simulink model "roll_1dof_model"  (R2024b)
settings: Solver=ode45  StartTime=0.0  StopTime=sim_stopTime  RelTol=1e-3
undefined symbols (not defined in the file): command_rollStep, command_stepTime, controller_inner_Kp, controller_outer_Kp, controller_outer_maxRateCmd, fin_actuatorTau, fin_maxDeflection, fin_maxRate, roll_design_Ixx, roll_design_p, roll_design_phi, roll_Ldelta, roll_Lp, sensor_attitudeTau, sensor_gyroTau
settings Model: Creator=kiwamoto  LastModifiedBy=kohei
settings ModelReferenceCC: UpdateModelReferenceTargets=IfOutOfDate

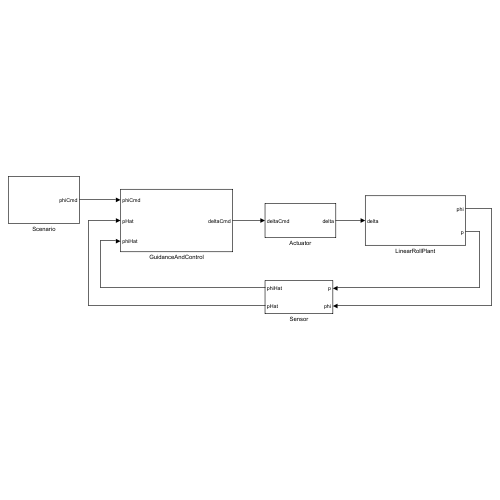
[thumbnail: Simulink's stored preview of the top-level diagram]
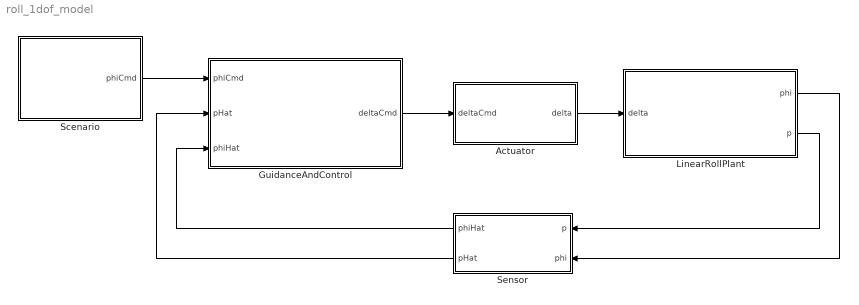
== system roll_1dof_model ==
  Actuator : Subsystem
  GuidanceAndControl : Subsystem
  LinearRollPlant : Subsystem
  Scenario : Subsystem
  Sensor : Subsystem
  wires:
  Scenario/1(phiCmd) -> GuidanceAndControl/1(phiCmd)
  GuidanceAndControl/1(deltaCmd) -> Actuator/1(deltaCmd)
  Actuator/1(delta) -> LinearRollPlant/1(delta)
  Sensor/1(phiHat) -> GuidanceAndControl/3(phiHat)
  Sensor/2(pHat) -> GuidanceAndControl/2(pHat)
  LinearRollPlant/2(p) -> Sensor/1(p)
  LinearRollPlant/1(phi) -> Sensor/2(phi)

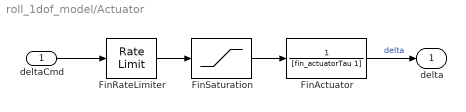
== system roll_1dof_model/Actuator ==
  deltaCmd : Inport
  FinActuator : TransferFcn  Denominator=[fin_actuatorTau 1]
  FinRateLimiter : RateLimiter  RisingSlewLimit=fin_maxRate  FallingSlewLimit=-fin_maxRate  SampleTimeMode=inherited
  FinSaturation : Saturate  UpperLimit=fin_maxDeflection  LowerLimit=-fin_maxDeflection
  delta : Outport
  wires:
  deltaCmd/1 -> FinRateLimiter/1
  FinRateLimiter/1 -> FinSaturation/1
  FinSaturation/1 -> FinActuator/1
  FinActuator/1 -> delta/1  "delta"

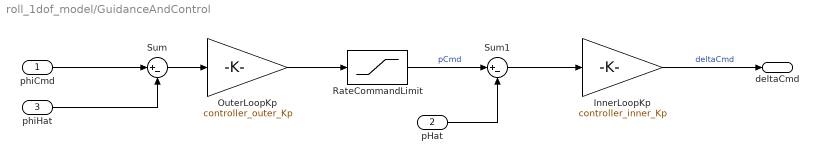
== system roll_1dof_model/GuidanceAndControl ==
  phiCmd : Inport
  pHat : Inport  Port=2
  phiHat : Inport  Port=3
  InnerLoopKp : Gain  Gain=controller_inner_Kp
  OuterLoopKp : Gain  Gain=controller_outer_Kp
  RateCommandLimit : Saturate  UpperLimit=controller_outer_maxRateCmd  LowerLimit=-controller_outer_maxRateCmd
  Sum : Sum  Inputs=|+-
  Sum1 : Sum  Inputs=|+-
  deltaCmd : Outport
  wires:
  phiCmd/1 -> Sum/1
  phiHat/1 -> Sum/2
  Sum/1 -> OuterLoopKp/1
  OuterLoopKp/1 -> RateCommandLimit/1
  pHat/1 -> Sum1/2
  Sum1/1 -> InnerLoopKp/1
  InnerLoopKp/1 -> deltaCmd/1  "deltaCmd"
  RateCommandLimit/1 -> Sum1/1  "pCmd"

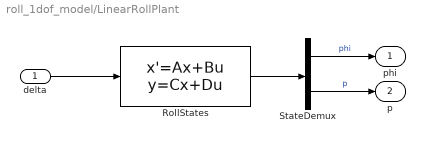
== system roll_1dof_model/LinearRollPlant ==
  delta : Inport
  RollStates : StateSpace  A=[0 1; 0 (roll_Lp)/(roll_design_Ixx)]  B=[0; (roll_Ldelta)/(roll_design_Ixx)]  C=eye(2)  D=[0; 0]  InitialCondition=[roll_design_phi; roll_design_p]
  StateDemux : Demux  Outputs=2
  phi : Outport
  p : Outport  Port=2
  wires:
  delta/1 -> RollStates/1
  RollStates/1 -> StateDemux/1
  StateDemux/2 -> p/1  "p"
  StateDemux/1 -> phi/1  "phi"

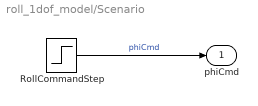
== system roll_1dof_model/Scenario ==
  RollCommandStep : Step  Time=command_stepTime  After=command_rollStep  SampleTime=0
  phiCmd : Outport
  wires:
  RollCommandStep/1 -> phiCmd/1  "phiCmd"

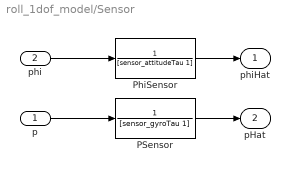
== system roll_1dof_model/Sensor ==
  p : Inport
  phi : Inport  Port=2
  PSensor : TransferFcn  Denominator=[sensor_gyroTau 1]
  PhiSensor : TransferFcn  Denominator=[sensor_attitudeTau 1]
  phiHat : Outport
  pHat : Outport  Port=2
  wires:
  PSensor/1 -> pHat/1
  phi/1 -> PhiSensor/1
  p/1 -> PSensor/1
  PhiSensor/1 -> phiHat/1
